simulink model "Control_simulacion_miercoles"  (R2016a)
settings: Solver=ode45  StartTime=0.0  StopTime=150  MaxStep=10e-3  RelTol=1e-3
values from neighbouring files (symbols this model uses):
  CLn = [1 0 0 ... (first row only)    [Control_MIMO_digital.m]
  DLn = [0 0 0 ... (first row only)    [Control_MIMO_digital.m]
  GLn = sysd.a    [Control_MIMO_digital.m]
  HLn = sysd.b    [Control_MIMO_digital.m]
  K = Grand*inv(X)    [Control_MIMO_digital.m]
  Kes = K(:,1:n)    [Control_MIMO_digital.m]
  Ki = -K(:,n+1:end)    [Control_MIMO_digital.m]
  Tm = 10e-3    (= 0.01)    [Control_MIMO_digital.m]
  u10 = double((a1*x20 + b1*x10^2)/u20)    [Control_MIMO_digital.m]
  u20 = double(sqrt(c1*x30*x20))    [Control_MIMO_digital.m]
  u30 = double((d1*x30 - u10)/x10)    [Control_MIMO_digital.m]
  x10 = 2    [Control_MIMO_digital.m]
  x20 = 4    [Control_MIMO_digital.m]
  x30 = 4    [Control_MIMO_digital.m]
  xini = [0.2; 0.6; 0.1]    [Control_MIMO_digital.m]
libraries: cstblocks x24
settings Model: Creator=Lenovo  LastModifiedBy=Lenovo

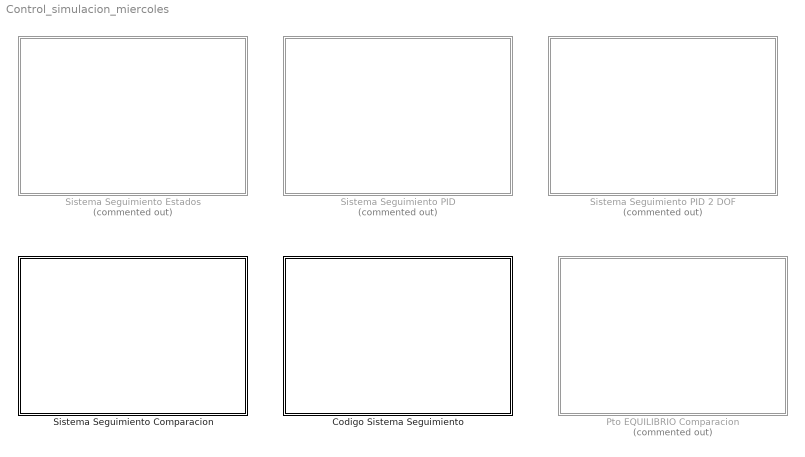
== system Control_simulacion_miercoles ==
  Codigo Sistema Seguimiento : Subsystem
  Pto EQUILIBRIO Comparacion : Subsystem  Commented=on
  Sistema Seguimiento Comparacion : Subsystem
  Sistema Seguimiento Estados : Subsystem  Commented=on
  Sistema Seguimiento PID : Subsystem  Commented=on
  Sistema Seguimiento PID 2 DOF : Subsystem  Commented=on

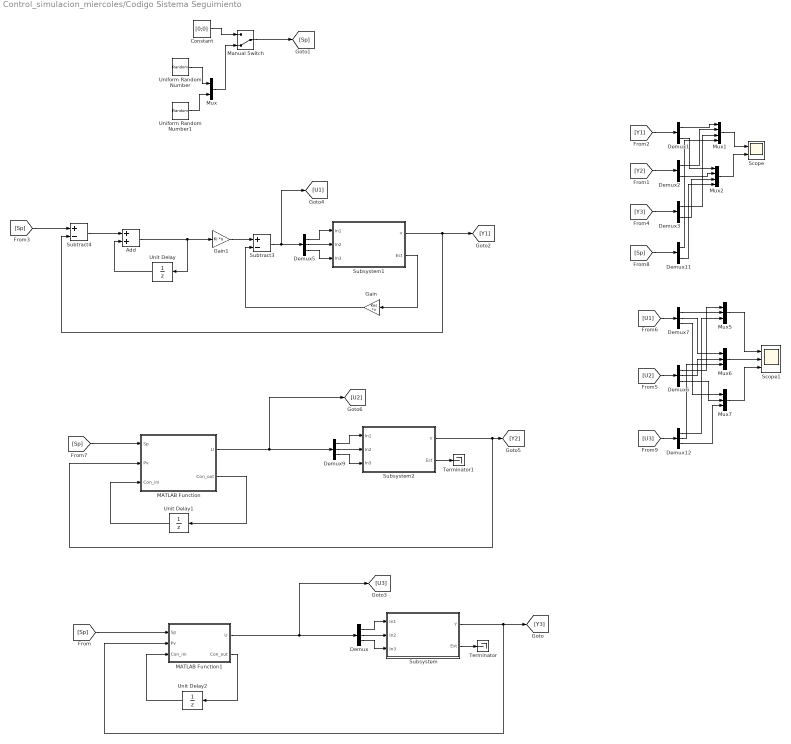
== system Control_simulacion_miercoles/Codigo Sistema Seguimiento ==
  Add : Sum
  Constant : Constant  Value=[0;0]
  Demux{,5..7,9,12} (6 alike) : Demux  Outputs=3
  Demux{1..3,11} (4 alike) : Demux  Outputs=2
  Gain : Gain  Gain=Kes  Multiplication=Matrix(K*u)
  Gain1 : Gain  Gain=Ki  Multiplication=Matrix(K*u)
  MATLAB Function : MATLAB Function  TreatAsAtomicUnit=on
  MATLAB Function1 : MATLAB Function  TreatAsAtomicUnit=on
  Manual Switch : ManualSwitch  CurrentSetting=0
  Mux : Mux  Inputs=2
  Mux1 : Mux
  Mux2 : Mux
  Mux5 : Mux  Inputs=3
  Mux6 : Mux  Inputs=3
  Mux7 : Mux  Inputs=3
  Scope : Scope  NumInputPorts=2
  Scope1 : Scope  NumInputPorts=3
  Subsystem : Subsystem
  Subsystem1 : Subsystem
  Subsystem2 : Subsystem
  Subtract3 : Sum  Inputs=+-
  Subtract4 : Sum  Inputs=+-
  Terminator : Terminator
  Terminator1 : Terminator
  Uniform Random Number : UniformRandomNumber  Minimum=-0.2  Maximum=0.2  SampleTime=3
  Uniform Random Number1 : UniformRandomNumber  Minimum=-0.4  Maximum=0.4  SampleTime=7
  Unit Delay : UnitDelay  SampleTime=Tm
  Unit Delay1 : UnitDelay  InitialCondition=zeros(4,1)  SampleTime=Tm
  Unit Delay2 : UnitDelay  InitialCondition=zeros(8,1)  SampleTime=Tm
  wires:
  Constant/1 -> Manual Switch/1
  Mux/1 -> Manual Switch/2
  Manual Switch/1 -> [Sp]
  Demux1/2 -> Mux2/1
  [Y1] -> Demux1/1
  [Y2] -> Demux2/1
  Demux2/1 -> Mux1/2
  Demux1/1 -> Mux1/1
  Demux2/2 -> Mux2/2
  Uniform Random Number1/1 -> Mux/2
  Uniform Random Number/1 -> Mux/1
  Demux/3 -> Subsystem/3(In3)
  Demux/2 -> Subsystem/2(In2)
  Demux/1 -> Subsystem/1(In1)
  Demux3/1 -> Mux1/3
  [Y3] -> Demux3/1
  Demux3/2 -> Mux2/3
  Mux2/1 -> Scope/2
  Mux1/1 -> Scope/1
  Subsystem/2(Est) -> Terminator/1
  [U2] -> Demux6/1
  [U1] -> Demux7/1
  Demux7/1 -> Mux5/1
  Demux6/1 -> Mux5/2
  Demux7/2 -> Mux6/1
  Demux6/2 -> Mux6/2
  Demux7/3 -> Mux7/1
  Demux6/3 -> Mux7/2
  Mux5/1 -> Scope1/1
  Mux6/1 -> Scope1/2
  Mux7/1 -> Scope1/3
  Subsystem/1(Y) -> MATLAB Function1/2(Pv), [Y3]
  MATLAB Function1/1(U) -> Demux/1, [U3]
  Demux5/3 -> Subsystem1/3(In3)
  Demux5/2 -> Subsystem1/2(In2)
  Demux5/1 -> Subsystem1/1(In1)
  Unit Delay/1 -> Add/2
  Subtract3/1 -> [U1], Demux5/1
  Subsystem1/1(Y) -> Subtract4/2, [Y1]
  Subtract4/1 -> Add/1
  Add/1 -> Unit Delay/1, Gain1/1
  Gain/1 -> Subtract3/2
  Gain1/1 -> Subtract3/1
  Subsystem1/2(Est) -> Gain/1
  [Sp] -> Subtract4/1
  Demux9/3 -> Subsystem2/3(In3)
  Demux9/2 -> Subsystem2/2(In2)
  Demux9/1 -> Subsystem2/1(In1)
  Subsystem2/1(Y) -> MATLAB Function/2(Pv), [Y2]
  Subsystem2/2(Est) -> Terminator1/1
  [Sp] -> Demux11/1
  Demux11/1 -> Mux1/4
  Demux11/2 -> Mux2/4
  [U3] -> Demux12/1
  Demux12/1 -> Mux5/3
  Demux12/2 -> Mux6/3
  Demux12/3 -> Mux7/3
  MATLAB Function/1(U) -> [U2], Demux9/1
  [Sp] -> MATLAB Function/1(Sp)
  Unit Delay1/1 -> MATLAB Function/3(Con_ini)
  MATLAB Function/2(Con_out) -> Unit Delay1/1
  [Sp] -> MATLAB Function1/1(Sp)
  Unit Delay2/1 -> MATLAB Function1/3(Con_ini)
  MATLAB Function1/2(Con_out) -> Unit Delay2/1

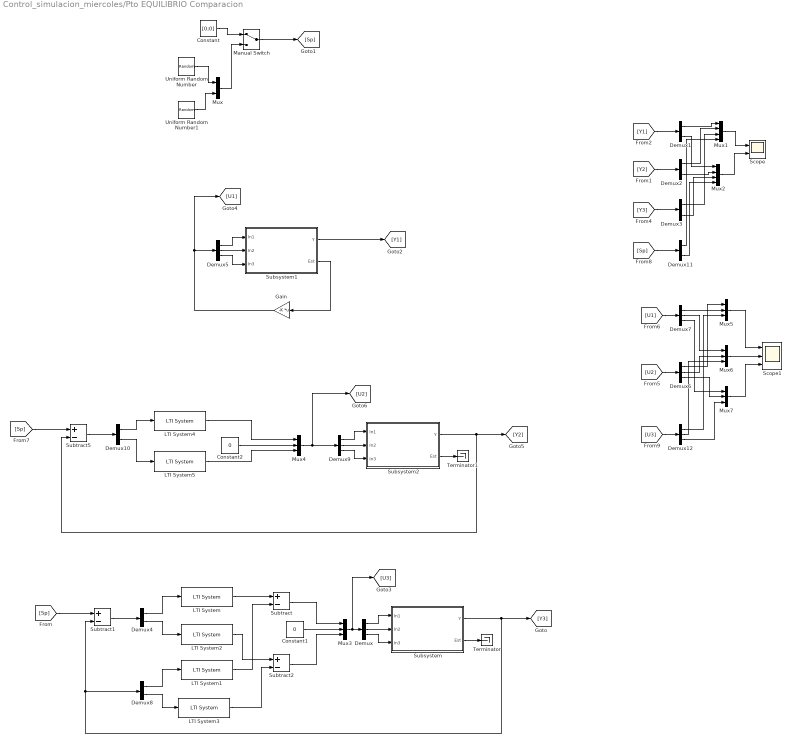
== system Control_simulacion_miercoles/Pto EQUILIBRIO Comparacion ==
  Constant : Constant  Value=[0;0]
  Constant1 : Constant  Value=0
  Constant2 : Constant  Value=0
  Demux{,5..7,9,12} (6 alike) : Demux  Outputs=3
  Demux{1..4,8,10..11} (7 alike) : Demux  Outputs=2
  Gain : Gain  Gain=-K  Multiplication=Matrix(K*u)
  LTI System : cstblocks/LTI System  sys=C11a  IC=[]
  LTI System1 : cstblocks/LTI System  sys=C11b  IC=[]
  LTI System2 : cstblocks/LTI System  sys=C23a  IC=[]
  LTI System3 : cstblocks/LTI System  sys=C23b  IC=[]
  LTI System4 : cstblocks/LTI System  sys=C11  IC=[]
  LTI System5 : cstblocks/LTI System  sys=C23  IC=[]
  Manual Switch : ManualSwitch
  Mux : Mux  Inputs=2
  Mux1 : Mux
  Mux2 : Mux
  Mux{3..7} (5 alike) : Mux  Inputs=3
  Scope : Scope  NumInputPorts=2
  Scope1 : Scope  NumInputPorts=3
  Subsystem : Subsystem
  Subsystem1 : Subsystem
  Subsystem2 : Subsystem
  Subtract{,1..2,5} (4 alike) : Sum  Inputs=+-
  Terminator : Terminator
  Terminator1 : Terminator
  Uniform Random Number : UniformRandomNumber  Minimum=-0.2  Maximum=0.2  SampleTime=3
  Uniform Random Number1 : UniformRandomNumber  Minimum=-0.4  Maximum=0.4  SampleTime=7
  wires:
  Constant/1 -> Manual Switch/1
  Mux/1 -> Manual Switch/2
  Manual Switch/1 -> [Sp]
  Demux1/2 -> Mux2/1
  [Y1] -> Demux1/1
  [Y2] -> Demux2/1
  Demux2/1 -> Mux1/2
  Demux1/1 -> Mux1/1
  Demux2/2 -> Mux2/2
  Uniform Random Number1/1 -> Mux/2
  Uniform Random Number/1 -> Mux/1
  Demux/3 -> Subsystem/3(In3)
  Demux/2 -> Subsystem/2(In2)
  Demux/1 -> Subsystem/1(In1)
  Demux3/1 -> Mux1/3
  [Y3] -> Demux3/1
  Demux3/2 -> Mux2/3
  Mux2/1 -> Scope/2
  Mux1/1 -> Scope/1
  [Sp] -> Subtract1/1
  Subsystem/2(Est) -> Terminator/1
  Subtract1/1 -> Demux4/1
  [U2] -> Demux6/1
  [U1] -> Demux7/1
  Demux7/1 -> Mux5/1
  Demux6/1 -> Mux5/2
  Demux7/2 -> Mux6/1
  Demux6/2 -> Mux6/2
  Demux7/3 -> Mux7/1
  Demux6/3 -> Mux7/2
  Mux5/1 -> Scope1/1
  Mux6/1 -> Scope1/2
  Mux7/1 -> Scope1/3
  Subsystem/1(Y) -> Subtract1/2, Demux8/1, [Y3]
  Demux4/1 -> LTI System/1
  Demux8/1 -> LTI System1/1
  LTI System/1 -> Subtract/1
  LTI System1/1 -> Subtract/2
  Demux4/2 -> LTI System2/1
  LTI System2/1 -> Subtract2/1
  Demux8/2 -> LTI System3/1
  LTI System3/1 -> Subtract2/2
  Mux3/1 -> [U3], Demux/1
  Subtract/1 -> Mux3/1
  Subtract2/1 -> Mux3/3
  Constant1/1 -> Mux3/2
  Demux5/3 -> Subsystem1/3(In3)
  Demux5/2 -> Subsystem1/2(In2)
  Demux5/1 -> Subsystem1/1(In1)
  Gain/1 -> [U1], Demux5/1
  Subsystem1/1(Y) -> [Y1]
  Subsystem1/2(Est) -> Gain/1
  Demux9/3 -> Subsystem2/3(In3)
  Demux9/2 -> Subsystem2/2(In2)
  Demux9/1 -> Subsystem2/1(In1)
  Subsystem2/1(Y) -> Subtract5/2, [Y2]
  [Sp] -> Subtract5/1
  Subsystem2/2(Est) -> Terminator1/1
  Subtract5/1 -> Demux10/1
  Demux10/1 -> LTI System4/1
  Demux10/2 -> LTI System5/1
  Mux4/1 -> [U2], Demux9/1
  LTI System4/1 -> Mux4/1
  LTI System5/1 -> Mux4/3
  Constant2/1 -> Mux4/2
  [Sp] -> Demux11/1
  Demux11/1 -> Mux1/4
  Demux11/2 -> Mux2/4
  [U3] -> Demux12/1
  Demux12/1 -> Mux5/3
  Demux12/2 -> Mux6/3
  Demux12/3 -> Mux7/3

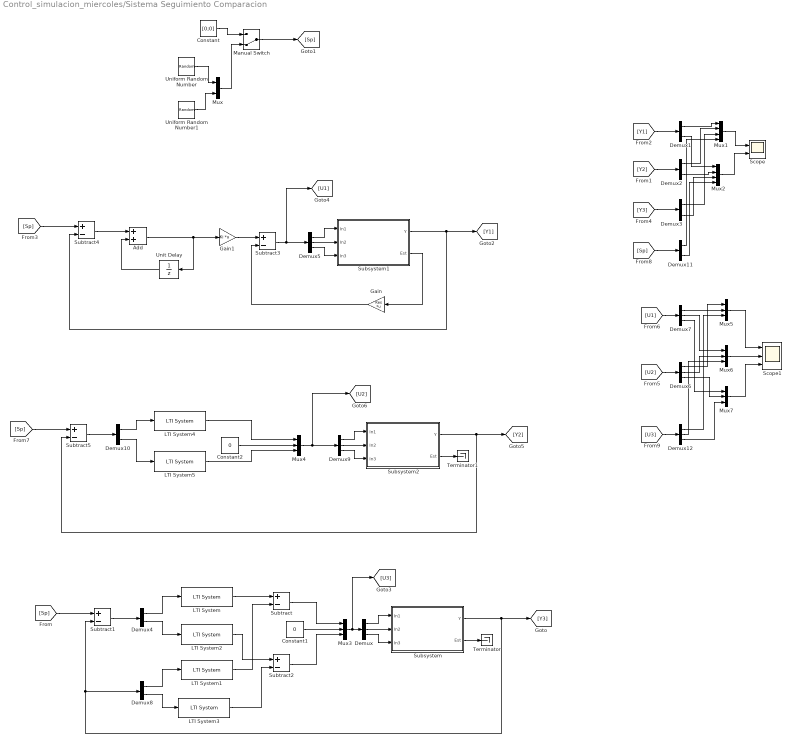
== system Control_simulacion_miercoles/Sistema Seguimiento Comparacion ==
  Add : Sum
  Constant : Constant  Value=[0;0]
  Constant1 : Constant  Value=0
  Constant2 : Constant  Value=0
  Demux{,5..7,9,12} (6 alike) : Demux  Outputs=3
  Demux{1..4,8,10..11} (7 alike) : Demux  Outputs=2
  Gain : Gain  Gain=Kes  Multiplication=Matrix(K*u)
  Gain1 : Gain  Gain=Ki  Multiplication=Matrix(K*u)
  LTI System : cstblocks/LTI System  sys=C11a  IC=[]
  LTI System1 : cstblocks/LTI System  sys=C11b  IC=[]
  LTI System2 : cstblocks/LTI System  sys=C23a  IC=[]
  LTI System3 : cstblocks/LTI System  sys=C23b  IC=[]
  LTI System4 : cstblocks/LTI System  sys=C11  IC=[]
  LTI System5 : cstblocks/LTI System  sys=C23  IC=[]
  Manual Switch : ManualSwitch  CurrentSetting=0
  Mux : Mux  Inputs=2
  Mux1 : Mux
  Mux2 : Mux
  Mux{3..7} (5 alike) : Mux  Inputs=3
  Scope : Scope  NumInputPorts=2
  Scope1 : Scope  NumInputPorts=3
  Subsystem : Subsystem
  Subsystem1 : Subsystem
  Subsystem2 : Subsystem
  Subtract{,1..5} (6 alike) : Sum  Inputs=+-
  Terminator : Terminator
  Terminator1 : Terminator
  Uniform Random Number : UniformRandomNumber  Minimum=-0.2  Maximum=0.2  SampleTime=3
  Uniform Random Number1 : UniformRandomNumber  Minimum=-0.4  Maximum=0.4  SampleTime=7
  Unit Delay : UnitDelay  SampleTime=Tm
  wires:
  Constant/1 -> Manual Switch/1
  Mux/1 -> Manual Switch/2
  Manual Switch/1 -> [Sp]
  Demux1/2 -> Mux2/1
  [Y1] -> Demux1/1
  [Y2] -> Demux2/1
  Demux2/1 -> Mux1/2
  Demux1/1 -> Mux1/1
  Demux2/2 -> Mux2/2
  Uniform Random Number1/1 -> Mux/2
  Uniform Random Number/1 -> Mux/1
  Demux/3 -> Subsystem/3(In3)
  Demux/2 -> Subsystem/2(In2)
  Demux/1 -> Subsystem/1(In1)
  Demux3/1 -> Mux1/3
  [Y3] -> Demux3/1
  Demux3/2 -> Mux2/3
  Mux2/1 -> Scope/2
  Mux1/1 -> Scope/1
  [Sp] -> Subtract1/1
  Subsystem/2(Est) -> Terminator/1
  Subtract1/1 -> Demux4/1
  [U2] -> Demux6/1
  [U1] -> Demux7/1
  Demux7/1 -> Mux5/1
  Demux6/1 -> Mux5/2
  Demux7/2 -> Mux6/1
  Demux6/2 -> Mux6/2
  Demux7/3 -> Mux7/1
  Demux6/3 -> Mux7/2
  Mux5/1 -> Scope1/1
  Mux6/1 -> Scope1/2
  Mux7/1 -> Scope1/3
  Subsystem/1(Y) -> Subtract1/2, Demux8/1, [Y3]
  Demux4/1 -> LTI System/1
  Demux8/1 -> LTI System1/1
  LTI System/1 -> Subtract/1
  LTI System1/1 -> Subtract/2
  Demux4/2 -> LTI System2/1
  LTI System2/1 -> Subtract2/1
  Demux8/2 -> LTI System3/1
  LTI System3/1 -> Subtract2/2
  Mux3/1 -> [U3], Demux/1
  Subtract/1 -> Mux3/1
  Subtract2/1 -> Mux3/3
  Constant1/1 -> Mux3/2
  Demux5/3 -> Subsystem1/3(In3)
  Demux5/2 -> Subsystem1/2(In2)
  Demux5/1 -> Subsystem1/1(In1)
  Unit Delay/1 -> Add/2
  Subtract3/1 -> [U1], Demux5/1
  Subsystem1/1(Y) -> Subtract4/2, [Y1]
  Subtract4/1 -> Add/1
  Add/1 -> Unit Delay/1, Gain1/1
  Gain/1 -> Subtract3/2
  Gain1/1 -> Subtract3/1
  Subsystem1/2(Est) -> Gain/1
  [Sp] -> Subtract4/1
  Demux9/3 -> Subsystem2/3(In3)
  Demux9/2 -> Subsystem2/2(In2)
  Demux9/1 -> Subsystem2/1(In1)
  Subsystem2/1(Y) -> Subtract5/2, [Y2]
  [Sp] -> Subtract5/1
  Subsystem2/2(Est) -> Terminator1/1
  Subtract5/1 -> Demux10/1
  Demux10/1 -> LTI System4/1
  Demux10/2 -> LTI System5/1
  Mux4/1 -> [U2], Demux9/1
  LTI System4/1 -> Mux4/1
  LTI System5/1 -> Mux4/3
  Constant2/1 -> Mux4/2
  [Sp] -> Demux11/1
  Demux11/1 -> Mux1/4
  Demux11/2 -> Mux2/4
  [U3] -> Demux12/1
  Demux12/1 -> Mux5/3
  Demux12/2 -> Mux6/3
  Demux12/3 -> Mux7/3

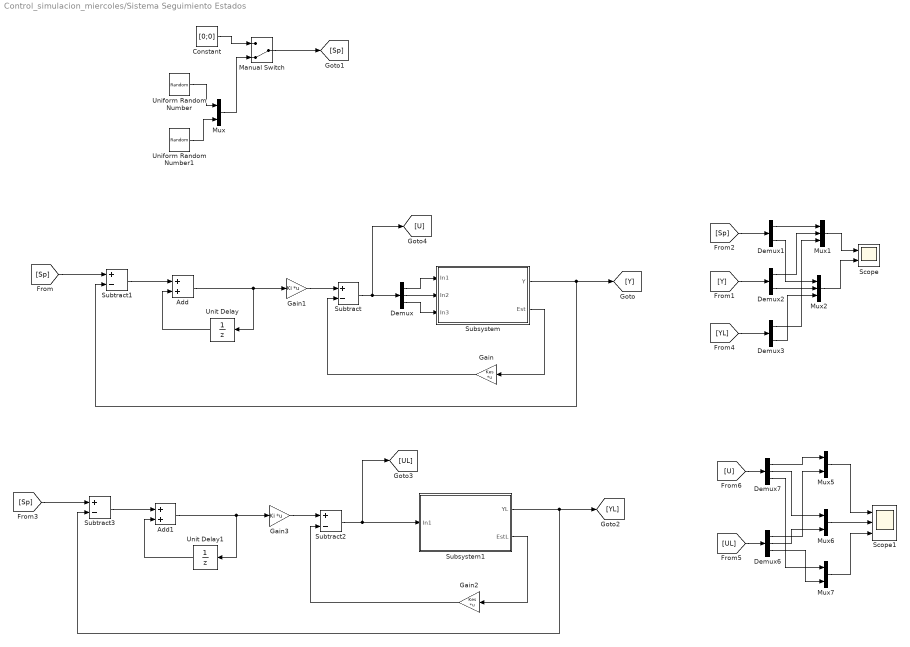
== system Control_simulacion_miercoles/Sistema Seguimiento Estados ==
  Add : Sum
  Add1 : Sum
  Constant : Constant  Value=[0;0]
  Demux : Demux  Outputs=3
  Demux1 : Demux  Outputs=2
  Demux2 : Demux  Outputs=2
  Demux3 : Demux  Outputs=2
  Demux6 : Demux  Outputs=3
  Demux7 : Demux  Outputs=3
  Gain : Gain  Gain=Kes  Multiplication=Matrix(K*u)
  Gain1 : Gain  Gain=Ki  Multiplication=Matrix(K*u)
  Gain2 : Gain  Gain=Kes  Multiplication=Matrix(K*u)
  Gain3 : Gain  Gain=Ki  Multiplication=Matrix(K*u)
  Manual Switch : ManualSwitch  CurrentSetting=0
  Mux{,5..7} (4 alike) : Mux  Inputs=2
  Mux1 : Mux  Inputs=3
  Mux2 : Mux  Inputs=3
  Scope : Scope  NumInputPorts=2
  Scope1 : Scope  NumInputPorts=3
  Subsystem : Subsystem
  Subsystem1 : Subsystem
  Subtract{,1..3} (4 alike) : Sum  Inputs=+-
  Uniform Random Number : UniformRandomNumber  Minimum=-0.2  Maximum=0.2  SampleTime=3
  Uniform Random Number1 : UniformRandomNumber  Minimum=-0.4  Maximum=0.4  SampleTime=7
  Unit Delay : UnitDelay  SampleTime=Tm
  Unit Delay1 : UnitDelay  SampleTime=Tm
  wires:
  Constant/1 -> Manual Switch/1
  Mux/1 -> Manual Switch/2
  Manual Switch/1 -> [Sp]
  Demux1/2 -> Mux2/1
  [Sp] -> Demux1/1
  [Y] -> Demux2/1
  Demux2/1 -> Mux1/2
  Demux1/1 -> Mux1/1
  Demux2/2 -> Mux2/2
  Uniform Random Number1/1 -> Mux/2
  Uniform Random Number/1 -> Mux/1
  Demux/3 -> Subsystem/3(In3)
  Demux/2 -> Subsystem/2(In2)
  Demux/1 -> Subsystem/1(In1)
  Unit Delay/1 -> Add/2
  Subtract/1 -> [U], Demux/1
  Demux3/1 -> Mux1/3
  Subsystem1/1(YL) -> Subtract3/2, [YL]
  Subsystem1/2(EstL) -> Gain2/1
  Gain3/1 -> Subtract2/1
  Add1/1 -> Unit Delay1/1, Gain3/1
  Unit Delay1/1 -> Add1/2
  Subtract3/1 -> Add1/1
  Gain2/1 -> Subtract2/2
  [Sp] -> Subtract3/1
  [YL] -> Demux3/1
  Subtract2/1 -> [UL], Subsystem1/1(In1)
  Demux3/2 -> Mux2/3
  Subsystem/1(Y) -> Subtract1/2, [Y]
  Subtract1/1 -> Add/1
  Add/1 -> Unit Delay/1, Gain1/1
  Mux2/1 -> Scope/2
  Mux1/1 -> Scope/1
  Gain/1 -> Subtract/2
  Gain1/1 -> Subtract/1
  Subsystem/2(Est) -> Gain/1
  [Sp] -> Subtract1/1
  [UL] -> Demux6/1
  [U] -> Demux7/1
  Demux7/1 -> Mux5/1
  Demux6/1 -> Mux5/2
  Demux7/2 -> Mux6/1
  Demux6/2 -> Mux6/2
  Demux7/3 -> Mux7/1
  Demux6/3 -> Mux7/2
  Mux5/1 -> Scope1/1
  Mux6/1 -> Scope1/2
  Mux7/1 -> Scope1/3

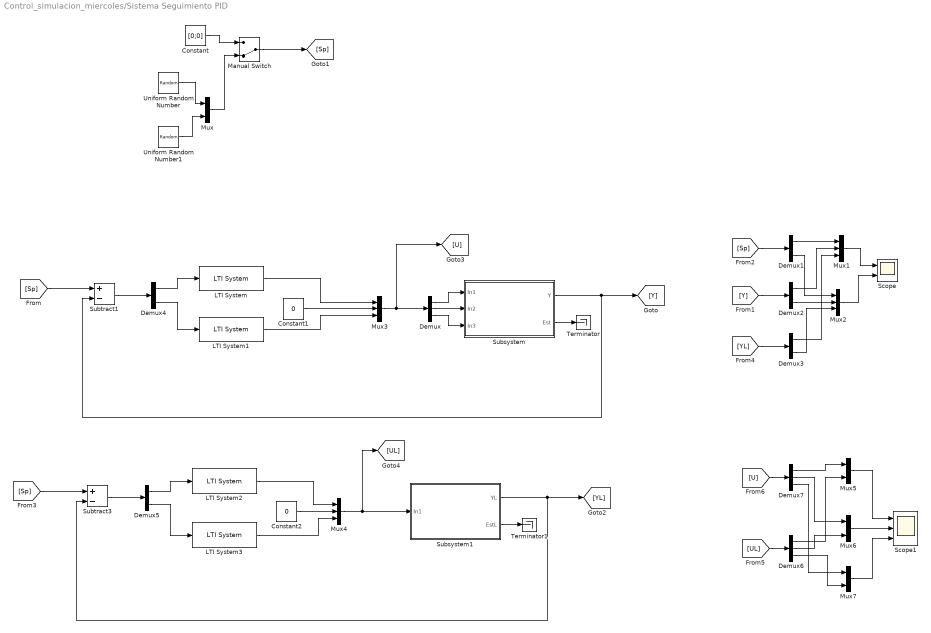
== system Control_simulacion_miercoles/Sistema Seguimiento PID ==
  Constant : Constant  Value=[0;0]
  Constant1 : Constant  Value=0
  Constant2 : Constant  Value=0
  Demux : Demux  Outputs=3
  Demux{1..5} (5 alike) : Demux  Outputs=2
  Demux6 : Demux  Outputs=3
  Demux7 : Demux  Outputs=3
  LTI System : cstblocks/LTI System  sys=C11  IC=[]
  LTI System1 : cstblocks/LTI System  sys=C23  IC=[]
  LTI System2 : cstblocks/LTI System  sys=C11  IC=[]
  LTI System3 : cstblocks/LTI System  sys=C23  IC=[]
  Manual Switch : ManualSwitch  CurrentSetting=0
  Mux{,5..7} (4 alike) : Mux  Inputs=2
  Mux{1..4} (4 alike) : Mux  Inputs=3
  Scope : Scope  NumInputPorts=2
  Scope1 : Scope  NumInputPorts=3
  Subsystem : Subsystem
  Subsystem1 : Subsystem
  Subtract1 : Sum  Inputs=+-
  Subtract3 : Sum  Inputs=+-
  Terminator : Terminator
  Terminator1 : Terminator
  Uniform Random Number : UniformRandomNumber  Minimum=-0.2  Maximum=0.2  SampleTime=3
  Uniform Random Number1 : UniformRandomNumber  Minimum=-0.4  Maximum=0.4  SampleTime=7
  wires:
  Constant/1 -> Manual Switch/1
  Mux/1 -> Manual Switch/2
  Manual Switch/1 -> [Sp]
  Demux1/2 -> Mux2/1
  [Sp] -> Demux1/1
  [Y] -> Demux2/1
  Demux2/1 -> Mux1/2
  Demux1/1 -> Mux1/1
  Demux2/2 -> Mux2/2
  Uniform Random Number1/1 -> Mux/2
  Uniform Random Number/1 -> Mux/1
  Demux/3 -> Subsystem/3(In3)
  Demux/2 -> Subsystem/2(In2)
  Demux/1 -> Subsystem/1(In1)
  Demux3/1 -> Mux1/3
  Subsystem1/1(YL) -> Subtract3/2, [YL]
  [Sp] -> Subtract3/1
  [YL] -> Demux3/1
  Demux3/2 -> Mux2/3
  Subsystem/1(Y) -> Subtract1/2, [Y]
  Mux2/1 -> Scope/2
  Mux1/1 -> Scope/1
  [Sp] -> Subtract1/1
  Subsystem/2(Est) -> Terminator/1
  Subtract1/1 -> Demux4/1
  Demux4/1 -> LTI System/1
  Demux4/2 -> LTI System1/1
  Mux3/1 -> [U], Demux/1
  LTI System/1 -> Mux3/1
  LTI System1/1 -> Mux3/3
  Constant1/1 -> Mux3/2
  Subsystem1/2(EstL) -> Terminator1/1
  Subtract3/1 -> Demux5/1
  Demux5/1 -> LTI System2/1
  Demux5/2 -> LTI System3/1
  LTI System2/1 -> Mux4/1
  LTI System3/1 -> Mux4/3
  Constant2/1 -> Mux4/2
  Mux4/1 -> [UL], Subsystem1/1(In1)
  [UL] -> Demux6/1
  [U] -> Demux7/1
  Demux7/1 -> Mux5/1
  Demux6/1 -> Mux5/2
  Demux7/2 -> Mux6/1
  Demux6/2 -> Mux6/2
  Demux7/3 -> Mux7/1
  Demux6/3 -> Mux7/2
  Mux5/1 -> Scope1/1
  Mux6/1 -> Scope1/2
  Mux7/1 -> Scope1/3

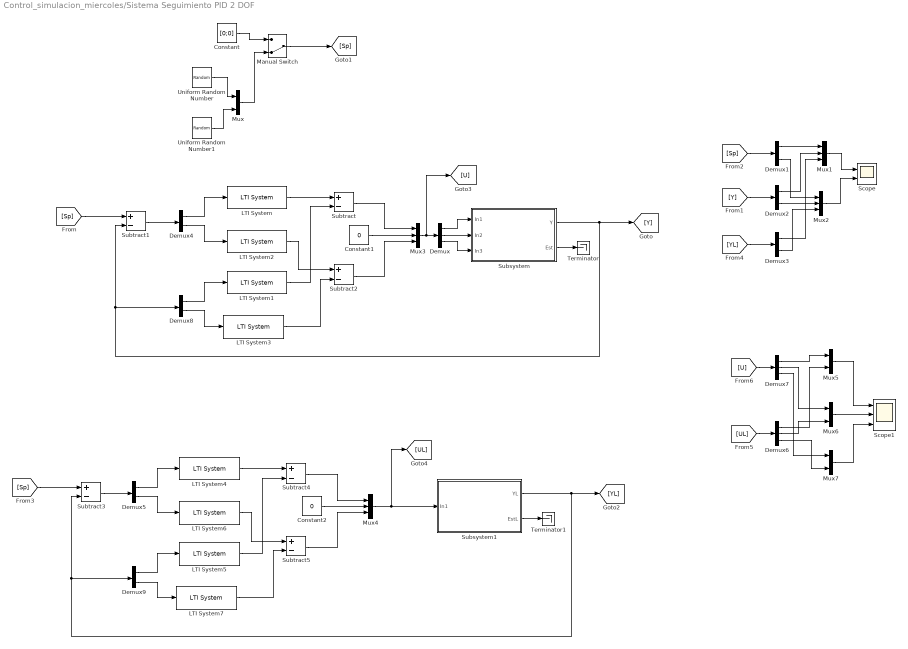
== system Control_simulacion_miercoles/Sistema Seguimiento PID 2 DOF ==
  Constant : Constant  Value=[0;0]
  Constant1 : Constant  Value=0
  Constant2 : Constant  Value=0
  Demux : Demux  Outputs=3
  Demux{1..5,8..9} (7 alike) : Demux  Outputs=2
  Demux6 : Demux  Outputs=3
  Demux7 : Demux  Outputs=3
  LTI System : cstblocks/LTI System  sys=C11a  IC=[]
  LTI System1 : cstblocks/LTI System  sys=C11b  IC=[]
  LTI System2 : cstblocks/LTI System  sys=C23a  IC=[]
  LTI System3 : cstblocks/LTI System  sys=C23b  IC=[]
  LTI System4 : cstblocks/LTI System  sys=C11a  IC=[]
  LTI System5 : cstblocks/LTI System  sys=C11b  IC=[]
  LTI System6 : cstblocks/LTI System  sys=C23a  IC=[]
  LTI System7 : cstblocks/LTI System  sys=C23b  IC=[]
  Manual Switch : ManualSwitch  CurrentSetting=0
  Mux{,5..7} (4 alike) : Mux  Inputs=2
  Mux{1..4} (4 alike) : Mux  Inputs=3
  Scope : Scope  NumInputPorts=2
  Scope1 : Scope  NumInputPorts=3
  Subsystem : Subsystem
  Subsystem1 : Subsystem
  Subtract{,1..5} (6 alike) : Sum  Inputs=+-
  Terminator : Terminator
  Terminator1 : Terminator
  Uniform Random Number : UniformRandomNumber  Minimum=-0.2  Maximum=0.2  SampleTime=3
  Uniform Random Number1 : UniformRandomNumber  Minimum=-0.4  Maximum=0.4  SampleTime=7
  wires:
  Constant/1 -> Manual Switch/1
  Mux/1 -> Manual Switch/2
  Manual Switch/1 -> [Sp]
  Demux1/2 -> Mux2/1
  [Sp] -> Demux1/1
  [Y] -> Demux2/1
  Demux2/1 -> Mux1/2
  Demux1/1 -> Mux1/1
  Demux2/2 -> Mux2/2
  Uniform Random Number1/1 -> Mux/2
  Uniform Random Number/1 -> Mux/1
  Demux/3 -> Subsystem/3(In3)
  Demux/2 -> Subsystem/2(In2)
  Demux/1 -> Subsystem/1(In1)
  Demux3/1 -> Mux1/3
  Subsystem1/1(YL) -> Demux9/1, Subtract3/2, [YL]
  [Sp] -> Subtract3/1
  [YL] -> Demux3/1
  Demux3/2 -> Mux2/3
  Mux2/1 -> Scope/2
  Mux1/1 -> Scope/1
  [Sp] -> Subtract1/1
  Subsystem/2(Est) -> Terminator/1
  Subtract1/1 -> Demux4/1
  Subsystem1/2(EstL) -> Terminator1/1
  [UL] -> Demux6/1
  [U] -> Demux7/1
  Demux7/1 -> Mux5/1
  Demux6/1 -> Mux5/2
  Demux7/2 -> Mux6/1
  Demux6/2 -> Mux6/2
  Demux7/3 -> Mux7/1
  Demux6/3 -> Mux7/2
  Mux5/1 -> Scope1/1
  Mux6/1 -> Scope1/2
  Mux7/1 -> Scope1/3
  Subsystem/1(Y) -> Subtract1/2, Demux8/1, [Y]
  Demux4/1 -> LTI System/1
  Demux8/1 -> LTI System1/1
  LTI System/1 -> Subtract/1
  LTI System1/1 -> Subtract/2
  Demux4/2 -> LTI System2/1
  LTI System2/1 -> Subtract2/1
  Demux8/2 -> LTI System3/1
  LTI System3/1 -> Subtract2/2
  Mux3/1 -> [U], Demux/1
  Subtract/1 -> Mux3/1
  Subtract2/1 -> Mux3/3
  Constant1/1 -> Mux3/2
  Subtract3/1 -> Demux5/1
  Demux5/1 -> LTI System4/1
  Demux9/1 -> LTI System5/1
  LTI System4/1 -> Subtract4/1
  LTI System5/1 -> Subtract4/2
  Demux5/2 -> LTI System6/1
  LTI System6/1 -> Subtract5/1
  Demux9/2 -> LTI System7/1
  LTI System7/1 -> Subtract5/2
  Subtract4/1 -> Mux4/1
  Subtract5/1 -> Mux4/3
  Constant2/1 -> Mux4/2
  Mux4/1 -> [UL], Subsystem1/1(In1)

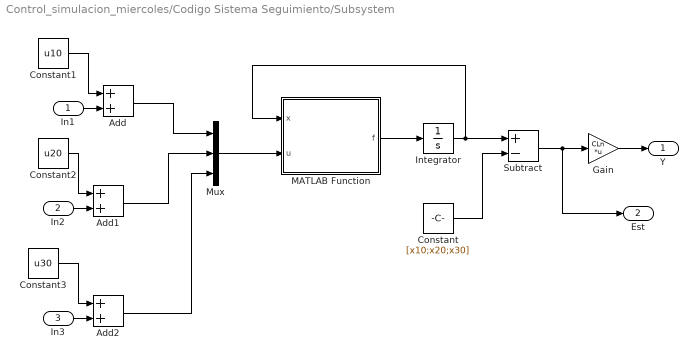
== system Control_simulacion_miercoles/Codigo Sistema Seguimiento/Subsystem ==
  In1 : Inport
  In2 : Inport  Port=2
  In3 : Inport  Port=3
  Add : Sum
  Add1 : Sum
  Add2 : Sum
  Constant : Constant  Value=[x10;x20;x30]
  Constant1 : Constant  Value=u10
  Constant2 : Constant  Value=u20
  Constant3 : Constant  Value=u30
  Gain : Gain  Gain=CLn  Multiplication=Matrix(K*u)
  Integrator : Integrator  InitialCondition=[x10;x20;x30]
  MATLAB Function : MATLAB Function  TreatAsAtomicUnit=on
  Mux : Mux  Inputs=3
  Subtract : Sum  Inputs=+-
  Y : Outport
  Est : Outport  Port=2
  wires:
  Add2/1 -> Mux/3
  Mux/1 -> MATLAB Function/2(u)
  Constant2/1 -> Add1/1
  Constant1/1 -> Add/1
  Constant3/1 -> Add2/1
  Integrator/1 -> MATLAB Function/1(x), Subtract/1
  Add/1 -> Mux/1
  Add1/1 -> Mux/2
  In2/1 -> Add1/2
  Gain/1 -> Y/1
  In1/1 -> Add/2
  In3/1 -> Add2/2
  MATLAB Function/1(f) -> Integrator/1
  Subtract/1 -> Est/1, Gain/1
  Constant/1 -> Subtract/2

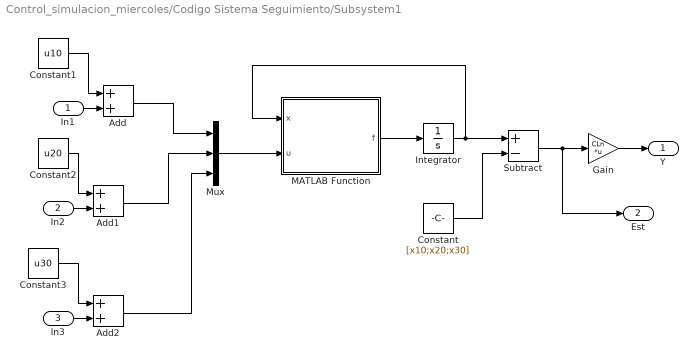
== system Control_simulacion_miercoles/Codigo Sistema Seguimiento/Subsystem1 ==
  In1 : Inport
  In2 : Inport  Port=2
  In3 : Inport  Port=3
  Add : Sum
  Add1 : Sum
  Add2 : Sum
  Constant : Constant  Value=[x10;x20;x30]
  Constant1 : Constant  Value=u10
  Constant2 : Constant  Value=u20
  Constant3 : Constant  Value=u30
  Gain : Gain  Gain=CLn  Multiplication=Matrix(K*u)
  Integrator : Integrator  InitialCondition=[x10;x20;x30]
  MATLAB Function : MATLAB Function  TreatAsAtomicUnit=on
  Mux : Mux  Inputs=3
  Subtract : Sum  Inputs=+-
  Y : Outport
  Est : Outport  Port=2
  wires:
  Add2/1 -> Mux/3
  Mux/1 -> MATLAB Function/2(u)
  Constant2/1 -> Add1/1
  Constant1/1 -> Add/1
  Constant3/1 -> Add2/1
  Integrator/1 -> MATLAB Function/1(x), Subtract/1
  Add/1 -> Mux/1
  Add1/1 -> Mux/2
  In2/1 -> Add1/2
  Gain/1 -> Y/1
  In1/1 -> Add/2
  In3/1 -> Add2/2
  MATLAB Function/1(f) -> Integrator/1
  Subtract/1 -> Est/1, Gain/1
  Constant/1 -> Subtract/2

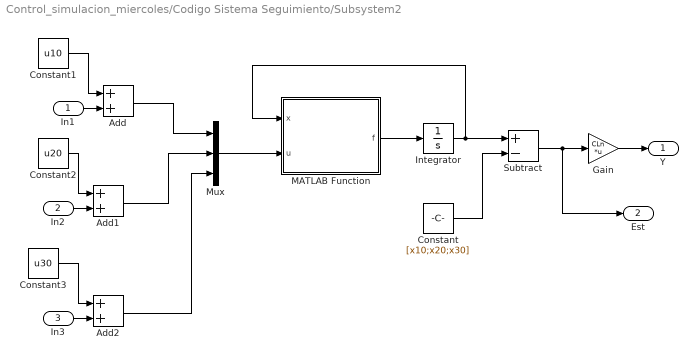
== system Control_simulacion_miercoles/Codigo Sistema Seguimiento/Subsystem2 ==
  In1 : Inport
  In2 : Inport  Port=2
  In3 : Inport  Port=3
  Add : Sum
  Add1 : Sum
  Add2 : Sum
  Constant : Constant  Value=[x10;x20;x30]
  Constant1 : Constant  Value=u10
  Constant2 : Constant  Value=u20
  Constant3 : Constant  Value=u30
  Gain : Gain  Gain=CLn  Multiplication=Matrix(K*u)
  Integrator : Integrator  InitialCondition=[x10;x20;x30]
  MATLAB Function : MATLAB Function  TreatAsAtomicUnit=on
  Mux : Mux  Inputs=3
  Subtract : Sum  Inputs=+-
  Y : Outport
  Est : Outport  Port=2
  wires:
  Add2/1 -> Mux/3
  Mux/1 -> MATLAB Function/2(u)
  Constant2/1 -> Add1/1
  Constant1/1 -> Add/1
  Constant3/1 -> Add2/1
  Integrator/1 -> MATLAB Function/1(x), Subtract/1
  Add/1 -> Mux/1
  Add1/1 -> Mux/2
  In2/1 -> Add1/2
  Gain/1 -> Y/1
  In1/1 -> Add/2
  In3/1 -> Add2/2
  MATLAB Function/1(f) -> Integrator/1
  Subtract/1 -> Est/1, Gain/1
  Constant/1 -> Subtract/2

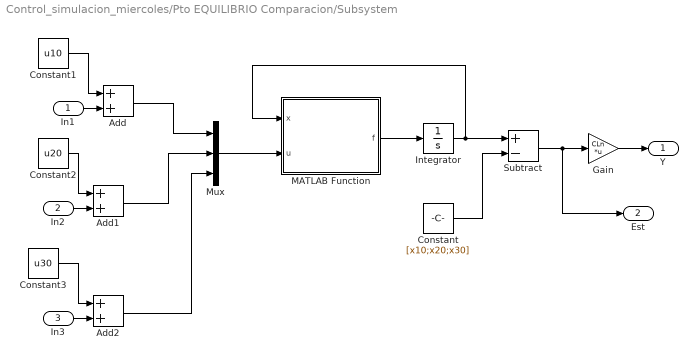
== system Control_simulacion_miercoles/Pto EQUILIBRIO Comparacion/Subsystem ==
  In1 : Inport
  In2 : Inport  Port=2
  In3 : Inport  Port=3
  Add : Sum
  Add1 : Sum
  Add2 : Sum
  Constant : Constant  Value=[x10;x20;x30]
  Constant1 : Constant  Value=u10
  Constant2 : Constant  Value=u20
  Constant3 : Constant  Value=u30
  Gain : Gain  Gain=CLn  Multiplication=Matrix(K*u)
  Integrator : Integrator  InitialCondition=[x10;x20;x30] + xini
  MATLAB Function : MATLAB Function  TreatAsAtomicUnit=on
  Mux : Mux  Inputs=3
  Subtract : Sum  Inputs=+-
  Y : Outport
  Est : Outport  Port=2
  wires:
  Add2/1 -> Mux/3
  Mux/1 -> MATLAB Function/2(u)
  Constant2/1 -> Add1/1
  Constant1/1 -> Add/1
  Constant3/1 -> Add2/1
  Integrator/1 -> MATLAB Function/1(x), Subtract/1
  Add/1 -> Mux/1
  Add1/1 -> Mux/2
  In2/1 -> Add1/2
  Gain/1 -> Y/1
  In1/1 -> Add/2
  In3/1 -> Add2/2
  MATLAB Function/1(f) -> Integrator/1
  Subtract/1 -> Est/1, Gain/1
  Constant/1 -> Subtract/2

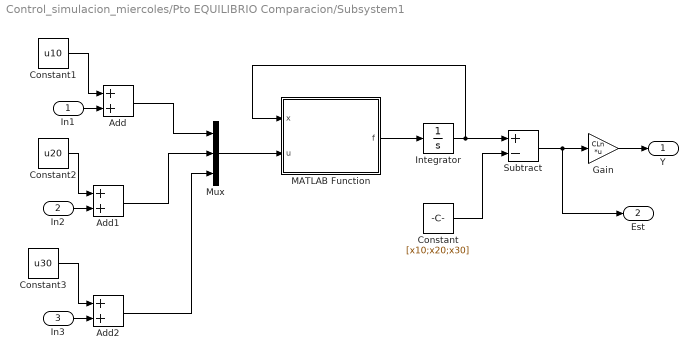
== system Control_simulacion_miercoles/Pto EQUILIBRIO Comparacion/Subsystem1 ==
  In1 : Inport
  In2 : Inport  Port=2
  In3 : Inport  Port=3
  Add : Sum
  Add1 : Sum
  Add2 : Sum
  Constant : Constant  Value=[x10;x20;x30]
  Constant1 : Constant  Value=u10
  Constant2 : Constant  Value=u20
  Constant3 : Constant  Value=u30
  Gain : Gain  Gain=CLn  Multiplication=Matrix(K*u)
  Integrator : Integrator  InitialCondition=[x10;x20;x30] + xini
  MATLAB Function : MATLAB Function  TreatAsAtomicUnit=on
  Mux : Mux  Inputs=3
  Subtract : Sum  Inputs=+-
  Y : Outport
  Est : Outport  Port=2
  wires:
  Add2/1 -> Mux/3
  Mux/1 -> MATLAB Function/2(u)
  Constant2/1 -> Add1/1
  Constant1/1 -> Add/1
  Constant3/1 -> Add2/1
  Integrator/1 -> MATLAB Function/1(x), Subtract/1
  Add/1 -> Mux/1
  Add1/1 -> Mux/2
  In2/1 -> Add1/2
  Gain/1 -> Y/1
  In1/1 -> Add/2
  In3/1 -> Add2/2
  MATLAB Function/1(f) -> Integrator/1
  Subtract/1 -> Est/1, Gain/1
  Constant/1 -> Subtract/2

== system Control_simulacion_miercoles/Pto EQUILIBRIO Comparacion/Subsystem2 ==
  In1 : Inport
  In2 : Inport  Port=2
  In3 : Inport  Port=3
  Add : Sum
  Add1 : Sum
  Add2 : Sum
  Constant : Constant  Value=[x10;x20;x30]
  Constant1 : Constant  Value=u10
  Constant2 : Constant  Value=u20
  Constant3 : Constant  Value=u30
  Gain : Gain  Gain=CLn  Multiplication=Matrix(K*u)
  Integrator : Integrator  InitialCondition=[x10;x20;x30] + xini
  MATLAB Function : MATLAB Function  TreatAsAtomicUnit=on
  Mux : Mux  Inputs=3
  Subtract : Sum  Inputs=+-
  Y : Outport
  Est : Outport  Port=2
  wires:
  Add2/1 -> Mux/3
  Mux/1 -> MATLAB Function/2(u)
  Constant2/1 -> Add1/1
  Constant1/1 -> Add/1
  Constant3/1 -> Add2/1
  Integrator/1 -> MATLAB Function/1(x), Subtract/1
  Add/1 -> Mux/1
  Add1/1 -> Mux/2
  In2/1 -> Add1/2
  Gain/1 -> Y/1
  In1/1 -> Add/2
  In3/1 -> Add2/2
  MATLAB Function/1(f) -> Integrator/1
  Subtract/1 -> Est/1, Gain/1
  Constant/1 -> Subtract/2

== system Control_simulacion_miercoles/Sistema Seguimiento Comparacion/Subsystem ==
  In1 : Inport
  In2 : Inport  Port=2
  In3 : Inport  Port=3
  Add : Sum
  Add1 : Sum
  Add2 : Sum
  Constant : Constant  Value=[x10;x20;x30]
  Constant1 : Constant  Value=u10
  Constant2 : Constant  Value=u20
  Constant3 : Constant  Value=u30
  Gain : Gain  Gain=CLn  Multiplication=Matrix(K*u)
  Integrator : Integrator  InitialCondition=[x10;x20;x30]
  MATLAB Function : MATLAB Function  TreatAsAtomicUnit=on
  Mux : Mux  Inputs=3
  Subtract : Sum  Inputs=+-
  Y : Outport
  Est : Outport  Port=2
  wires:
  Add2/1 -> Mux/3
  Mux/1 -> MATLAB Function/2(u)
  Constant2/1 -> Add1/1
  Constant1/1 -> Add/1
  Constant3/1 -> Add2/1
  Integrator/1 -> MATLAB Function/1(x), Subtract/1
  Add/1 -> Mux/1
  Add1/1 -> Mux/2
  In2/1 -> Add1/2
  Gain/1 -> Y/1
  In1/1 -> Add/2
  In3/1 -> Add2/2
  MATLAB Function/1(f) -> Integrator/1
  Subtract/1 -> Est/1, Gain/1
  Constant/1 -> Subtract/2

== system Control_simulacion_miercoles/Sistema Seguimiento Comparacion/Subsystem1 ==
  In1 : Inport
  In2 : Inport  Port=2
  In3 : Inport  Port=3
  Add : Sum
  Add1 : Sum
  Add2 : Sum
  Constant : Constant  Value=[x10;x20;x30]
  Constant1 : Constant  Value=u10
  Constant2 : Constant  Value=u20
  Constant3 : Constant  Value=u30
  Gain : Gain  Gain=CLn  Multiplication=Matrix(K*u)
  Integrator : Integrator  InitialCondition=[x10;x20;x30]
  MATLAB Function : MATLAB Function  TreatAsAtomicUnit=on
  Mux : Mux  Inputs=3
  Subtract : Sum  Inputs=+-
  Y : Outport
  Est : Outport  Port=2
  wires:
  Add2/1 -> Mux/3
  Mux/1 -> MATLAB Function/2(u)
  Constant2/1 -> Add1/1
  Constant1/1 -> Add/1
  Constant3/1 -> Add2/1
  Integrator/1 -> MATLAB Function/1(x), Subtract/1
  Add/1 -> Mux/1
  Add1/1 -> Mux/2
  In2/1 -> Add1/2
  Gain/1 -> Y/1
  In1/1 -> Add/2
  In3/1 -> Add2/2
  MATLAB Function/1(f) -> Integrator/1
  Subtract/1 -> Est/1, Gain/1
  Constant/1 -> Subtract/2

== system Control_simulacion_miercoles/Sistema Seguimiento Comparacion/Subsystem2 ==
  In1 : Inport
  In2 : Inport  Port=2
  In3 : Inport  Port=3
  Add : Sum
  Add1 : Sum
  Add2 : Sum
  Constant : Constant  Value=[x10;x20;x30]
  Constant1 : Constant  Value=u10
  Constant2 : Constant  Value=u20
  Constant3 : Constant  Value=u30
  Gain : Gain  Gain=CLn  Multiplication=Matrix(K*u)
  Integrator : Integrator  InitialCondition=[x10;x20;x30]
  MATLAB Function : MATLAB Function  TreatAsAtomicUnit=on
  Mux : Mux  Inputs=3
  Subtract : Sum  Inputs=+-
  Y : Outport
  Est : Outport  Port=2
  wires:
  Add2/1 -> Mux/3
  Mux/1 -> MATLAB Function/2(u)
  Constant2/1 -> Add1/1
  Constant1/1 -> Add/1
  Constant3/1 -> Add2/1
  Integrator/1 -> MATLAB Function/1(x), Subtract/1
  Add/1 -> Mux/1
  Add1/1 -> Mux/2
  In2/1 -> Add1/2
  Gain/1 -> Y/1
  In1/1 -> Add/2
  In3/1 -> Add2/2
  MATLAB Function/1(f) -> Integrator/1
  Subtract/1 -> Est/1, Gain/1
  Constant/1 -> Subtract/2

== system Control_simulacion_miercoles/Sistema Seguimiento Estados/Subsystem ==
  In1 : Inport
  In2 : Inport  Port=2
  In3 : Inport  Port=3
  Add : Sum
  Add1 : Sum
  Add2 : Sum
  Constant : Constant  Value=[x10;x20;x30]
  Constant1 : Constant  Value=u10
  Constant2 : Constant  Value=u20
  Constant3 : Constant  Value=u30
  Gain : Gain  Gain=CLn  Multiplication=Matrix(K*u)
  Integrator : Integrator  InitialCondition=[x10;x20;x30]
  MATLAB Function : MATLAB Function  TreatAsAtomicUnit=on
  Mux : Mux  Inputs=3
  Subtract : Sum  Inputs=+-
  Y : Outport
  Est : Outport  Port=2
  wires:
  Add2/1 -> Mux/3
  Mux/1 -> MATLAB Function/2(u)
  Constant2/1 -> Add1/1
  Constant1/1 -> Add/1
  Constant3/1 -> Add2/1
  Integrator/1 -> MATLAB Function/1(x), Subtract/1
  Add/1 -> Mux/1
  Add1/1 -> Mux/2
  In2/1 -> Add1/2
  Gain/1 -> Y/1
  In1/1 -> Add/2
  In3/1 -> Add2/2
  MATLAB Function/1(f) -> Integrator/1
  Subtract/1 -> Est/1, Gain/1
  Constant/1 -> Subtract/2

== system Control_simulacion_miercoles/Sistema Seguimiento Estados/Subsystem1 ==
  In1 : Inport
  Add : Sum
  Add3 : Sum
  Gain : Gain  Gain=CLn  Multiplication=Matrix(K*u)
  Gain1 : Gain  Gain=GLn  Multiplication=Matrix(K*u)
  Gain2 : Gain  Gain=DLn  Multiplication=Matrix(K*u)
  Gain3 : Gain  Gain=HLn  Multiplication=Matrix(K*u)
  Unit Delay : UnitDelay  SampleTime=Tm
  YL : Outport
  EstL : Outport  Port=2
  wires:
  Add/1 -> Unit Delay/1
  Gain1/1 -> Add/2
  Unit Delay/1 -> Gain/1, EstL/1, Gain1/1
  Gain/1 -> Add3/2
  Add3/1 -> YL/1
  Gain2/1 -> Add3/1
  Gain3/1 -> Add/1
  In1/1 -> Gain2/1, Gain3/1

== system Control_simulacion_miercoles/Sistema Seguimiento PID/Subsystem ==
  In1 : Inport
  In2 : Inport  Port=2
  In3 : Inport  Port=3
  Add : Sum
  Add1 : Sum
  Add2 : Sum
  Constant : Constant  Value=[x10;x20;x30]
  Constant1 : Constant  Value=u10
  Constant2 : Constant  Value=u20
  Constant3 : Constant  Value=u30
  Gain : Gain  Gain=CLn  Multiplication=Matrix(K*u)
  Integrator : Integrator  InitialCondition=[x10;x20;x30]
  MATLAB Function : MATLAB Function  TreatAsAtomicUnit=on
  Mux : Mux  Inputs=3
  Subtract : Sum  Inputs=+-
  Y : Outport
  Est : Outport  Port=2
  wires:
  Add2/1 -> Mux/3
  Mux/1 -> MATLAB Function/2(u)
  Constant2/1 -> Add1/1
  Constant1/1 -> Add/1
  Constant3/1 -> Add2/1
  Integrator/1 -> MATLAB Function/1(x), Subtract/1
  Add/1 -> Mux/1
  Add1/1 -> Mux/2
  In2/1 -> Add1/2
  Gain/1 -> Y/1
  In1/1 -> Add/2
  In3/1 -> Add2/2
  MATLAB Function/1(f) -> Integrator/1
  Subtract/1 -> Est/1, Gain/1
  Constant/1 -> Subtract/2

== system Control_simulacion_miercoles/Sistema Seguimiento PID/Subsystem1 ==
  In1 : Inport
  Add : Sum
  Add3 : Sum
  Gain : Gain  Gain=CLn  Multiplication=Matrix(K*u)
  Gain1 : Gain  Gain=GLn  Multiplication=Matrix(K*u)
  Gain2 : Gain  Gain=DLn  Multiplication=Matrix(K*u)
  Gain3 : Gain  Gain=HLn  Multiplication=Matrix(K*u)
  Unit Delay : UnitDelay  SampleTime=Tm
  YL : Outport
  EstL : Outport  Port=2
  wires:
  Add/1 -> Unit Delay/1
  Gain1/1 -> Add/2
  Unit Delay/1 -> Gain/1, EstL/1, Gain1/1
  Gain/1 -> Add3/2
  Add3/1 -> YL/1
  Gain2/1 -> Add3/1
  Gain3/1 -> Add/1
  In1/1 -> Gain2/1, Gain3/1

== system Control_simulacion_miercoles/Sistema Seguimiento PID 2 DOF/Subsystem ==
  In1 : Inport
  In2 : Inport  Port=2
  In3 : Inport  Port=3
  Add : Sum
  Add1 : Sum
  Add2 : Sum
  Constant : Constant  Value=[x10;x20;x30]
  Constant1 : Constant  Value=u10
  Constant2 : Constant  Value=u20
  Constant3 : Constant  Value=u30
  Gain : Gain  Gain=CLn  Multiplication=Matrix(K*u)
  Integrator : Integrator  InitialCondition=[x10;x20;x30]
  MATLAB Function : MATLAB Function  TreatAsAtomicUnit=on
  Mux : Mux  Inputs=3
  Subtract : Sum  Inputs=+-
  Y : Outport
  Est : Outport  Port=2
  wires:
  Add2/1 -> Mux/3
  Mux/1 -> MATLAB Function/2(u)
  Constant2/1 -> Add1/1
  Constant1/1 -> Add/1
  Constant3/1 -> Add2/1
  Integrator/1 -> MATLAB Function/1(x), Subtract/1
  Add/1 -> Mux/1
  Add1/1 -> Mux/2
  In2/1 -> Add1/2
  Gain/1 -> Y/1
  In1/1 -> Add/2
  In3/1 -> Add2/2
  MATLAB Function/1(f) -> Integrator/1
  Subtract/1 -> Est/1, Gain/1
  Constant/1 -> Subtract/2

== system Control_simulacion_miercoles/Sistema Seguimiento PID 2 DOF/Subsystem1 ==
  In1 : Inport
  Add : Sum
  Add3 : Sum
  Gain : Gain  Gain=CLn  Multiplication=Matrix(K*u)
  Gain1 : Gain  Gain=GLn  Multiplication=Matrix(K*u)
  Gain2 : Gain  Gain=DLn  Multiplication=Matrix(K*u)
  Gain3 : Gain  Gain=HLn  Multiplication=Matrix(K*u)
  Unit Delay : UnitDelay  SampleTime=Tm
  YL : Outport
  EstL : Outport  Port=2
  wires:
  Add/1 -> Unit Delay/1
  Gain1/1 -> Add/2
  Unit Delay/1 -> Gain/1, EstL/1, Gain1/1
  Gain/1 -> Add3/2
  Add3/1 -> YL/1
  Gain2/1 -> Add3/1
  Gain3/1 -> Add/1
  In1/1 -> Gain2/1, Gain3/1

== matlab function Control_simulacion_miercoles/Sistema Seguimiento PID/Subsystem/MATLAB Function ==
  data: x input; u input; f output
function f = fcn(x,u)

a = 2;
b = 4;
c = 1;
d = 3;

x1 = x(1);
x2 = x(2);
x3 = x(3);
u1 = u(1);
u2 = u(2);
u3 = u(3);
f1 = -a*x2 - b*x1^2 + u1*u2;
f2 = -c*x3*x2 + u2^2 ;
f3 = -d*x3 + u3*x1 + u1;
f = [f1; f2; f3];

== matlab function Control_simulacion_miercoles/Sistema Seguimiento Estados/Subsystem/MATLAB Function ==
  data: x input; u input; f output
function f = fcn(x,u)

a = 2;
b = 4;
c = 1;
d = 3;

x1 = x(1);
x2 = x(2);
x3 = x(3);
u1 = u(1);
u2 = u(2);
u3 = u(3);
f1 = -a*x2 - b*x1^2 + u1*u2;
f2 = -c*x3*x2 + u2^2 ;
f3 = -d*x3 + u3*x1 + u1;
f = [f1; f2; f3];

== matlab function Control_simulacion_miercoles/Sistema Seguimiento PID 2 DOF/Subsystem/MATLAB Function ==
  data: x input; u input; f output
function f = fcn(x,u)

a = 2;
b = 4;
c = 1;
d = 3;

x1 = x(1);
x2 = x(2);
x3 = x(3);
u1 = u(1);
u2 = u(2);
u3 = u(3);
f1 = -a*x2 - b*x1^2 + u1*u2;
f2 = -c*x3*x2 + u2^2 ;
f3 = -d*x3 + u3*x1 + u1;
f = [f1; f2; f3];

== matlab function Control_simulacion_miercoles/Sistema Seguimiento Comparacion/Subsystem/MATLAB Function ==
  data: x input; u input; f output
function f = fcn(x,u)

a = 2;
b = 4;
c = 1;
d = 3;

x1 = x(1);
x2 = x(2);
x3 = x(3);
u1 = u(1);
u2 = u(2);
u3 = u(3);
f1 = -a*x2 - b*x1^2 + u1*u2;
f2 = -c*x3*x2 + u2^2 ;
f3 = -d*x3 + u3*x1 + u1;
f = [f1; f2; f3];

== matlab function Control_simulacion_miercoles/Sistema Seguimiento Comparacion/Subsystem1/MATLAB Function ==
  data: x input; u input; f output
function f = fcn(x,u)

a = 2;
b = 4;
c = 1;
d = 3;

x1 = x(1);
x2 = x(2);
x3 = x(3);
u1 = u(1);
u2 = u(2);
u3 = u(3);
f1 = -a*x2 - b*x1^2 + u1*u2;
f2 = -c*x3*x2 + u2^2 ;
f3 = -d*x3 + u3*x1 + u1;
f = [f1; f2; f3];

== matlab function Control_simulacion_miercoles/Sistema Seguimiento Comparacion/Subsystem2/MATLAB Function ==
  data: x input; u input; f output
function f = fcn(x,u)

a = 2;
b = 4;
c = 1;
d = 3;

x1 = x(1);
x2 = x(2);
x3 = x(3);
u1 = u(1);
u2 = u(2);
u3 = u(3);
f1 = -a*x2 - b*x1^2 + u1*u2;
f2 = -c*x3*x2 + u2^2 ;
f3 = -d*x3 + u3*x1 + u1;
f = [f1; f2; f3];

== matlab function Control_simulacion_miercoles/Pto EQUILIBRIO Comparacion/Subsystem/MATLAB Function ==
  data: x input; u input; f output
function f = fcn(x,u)

a = 2;
b = 4;
c = 1;
d = 3;

x1 = x(1);
x2 = x(2);
x3 = x(3);
u1 = u(1);
u2 = u(2);
u3 = u(3);
f1 = -a*x2 - b*x1^2 + u1*u2;
f2 = -c*x3*x2 + u2^2 ;
f3 = -d*x3 + u3*x1 + u1;
f = [f1; f2; f3];

== matlab function Control_simulacion_miercoles/Pto EQUILIBRIO Comparacion/Subsystem1/MATLAB Function ==
  data: x input; u input; f output
function f = fcn(x,u)

a = 2;
b = 4;
c = 1;
d = 3;

x1 = x(1);
x2 = x(2);
x3 = x(3);
u1 = u(1);
u2 = u(2);
u3 = u(3);
f1 = -a*x2 - b*x1^2 + u1*u2;
f2 = -c*x3*x2 + u2^2 ;
f3 = -d*x3 + u3*x1 + u1;
f = [f1; f2; f3];

== matlab function Control_simulacion_miercoles/Pto EQUILIBRIO Comparacion/Subsystem2/MATLAB Function ==
  data: x input; u input; f output
function f = fcn(x,u)

a = 2;
b = 4;
c = 1;
d = 3;

x1 = x(1);
x2 = x(2);
x3 = x(3);
u1 = u(1);
u2 = u(2);
u3 = u(3);
f1 = -a*x2 - b*x1^2 + u1*u2;
f2 = -c*x3*x2 + u2^2 ;
f3 = -d*x3 + u3*x1 + u1;
f = [f1; f2; f3];

== matlab function Control_simulacion_miercoles/Codigo Sistema Seguimiento/Subsystem/MATLAB Function ==
  data: x input; u input; f output
function f = fcn(x,u)

a = 2;
b = 4;
c = 1;
d = 3;

x1 = x(1);
x2 = x(2);
x3 = x(3);
u1 = u(1);
u2 = u(2);
u3 = u(3);
f1 = -a*x2 - b*x1^2 + u1*u2;
f2 = -c*x3*x2 + u2^2 ;
f3 = -d*x3 + u3*x1 + u1;
f = [f1; f2; f3];

== matlab function Control_simulacion_miercoles/Codigo Sistema Seguimiento/Subsystem1/MATLAB Function ==
  data: x input; u input; f output
function f = fcn(x,u)

a = 2;
b = 4;
c = 1;
d = 3;

x1 = x(1);
x2 = x(2);
x3 = x(3);
u1 = u(1);
u2 = u(2);
u3 = u(3);
f1 = -a*x2 - b*x1^2 + u1*u2;
f2 = -c*x3*x2 + u2^2 ;
f3 = -d*x3 + u3*x1 + u1;
f = [f1; f2; f3];

== matlab function Control_simulacion_miercoles/Codigo Sistema Seguimiento/Subsystem2/MATLAB Function ==
  data: x input; u input; f output
function f = fcn(x,u)

a = 2;
b = 4;
c = 1;
d = 3;

x1 = x(1);
x2 = x(2);
x3 = x(3);
u1 = u(1);
u2 = u(2);
u3 = u(3);
f1 = -a*x2 - b*x1^2 + u1*u2;
f2 = -c*x3*x2 + u2^2 ;
f3 = -d*x3 + u3*x1 + u1;
f = [f1; f2; f3];

== matlab function Control_simulacion_miercoles/Codigo Sistema Seguimiento/MATLAB Function ==
  data: Sp input; U output; Pv input; Con_ini input; Con_out output
function [U,Con_out] = fcn(Sp,Pv,Con_ini)

e1_1 = Con_ini(1);
u1_1 = Con_ini(2);
e2_1 = Con_ini(3);
u2_1 = Con_ini(4);

Sp1 = Sp(1);
Pv1 = Pv(1);
e1 = Sp1-Pv1; 
u1 = 2*e1 - 1.68*e1_1 + u1_1;
e1_1 = e1;
u1_1 = u1;

Sp2 = Sp(2);
Pv2 = Pv(2);
e2 = Sp2-Pv2; 
u2 = 7*e2 - 5.6*e2_1 + u2_1;
e2_1 = e2;
u2_1 = u2;

U = [u1;0;u2];
Con_out = [e1_1; u1_1; e2_1; u2_1];

== matlab function Control_simulacion_miercoles/Codigo Sistema Seguimiento/MATLAB Function1 ==
  data: Sp input; U output; Pv input; Con_ini input; Con_out output
function [U,Con_out] = fcn(Sp,Pv,Con_ini)

e1_1 = Con_ini(1);
u1a_1 = Con_ini(2);
Pv1_1 = Con_ini(3);
u1b_1 = Con_ini(4);
e2_1 = Con_ini(5);
u2a_1 = Con_ini(6);
Pv2_1 = Con_ini(7);
u2b_1 = Con_ini(8);

Sp1 = Sp(1);
Pv1 = Pv(1);
e1 = Sp1-Pv1;
u1a = 6.8*e1 - 5.78*e1_1 + u1a_1;
u1b = 0.07*Pv1 - 0.0539*Pv1_1 + 0.93*u1b_1;
u1 = u1a - u1b;
e1_1 = e1;
u1a_1 = u1a;
Pv1_1 = Pv1;
u1b_1 = u1b;


Sp2 = Sp(2);
Pv2 = Pv(2);
e2 = Sp2-Pv2;
u2a = 2.5*e2 - 1.5*e2_1 + u2a_1;
u2b = 4*Pv2 - 1.6*Pv2_1 + 0.8*u2b_1;
u2 = u2a - u2b;

e2_1 = e2;
u2a_1 = u2a;
Pv2_1 = Pv2;
u2b_1 = u2b;

U = [u1;0;u2];

Con_out = [e1_1; u1a_1; Pv1_1; u1b_1; e2_1; u2a_1; Pv2_1; u2b_1];
